simulink model "Hopper_3DOF"  (R2025a)
settings: Solver=FixedStepAuto  StartTime=0.0  StopTime=10  FixedStep=0.05  RelTol=1e-3
model workspace (MAT data in the model file):
  Inertia = 5000
  Prop_Mass = 50
libraries: aerolibanim x1
settings Model: Creator=asing  LastModifiedBy=asing

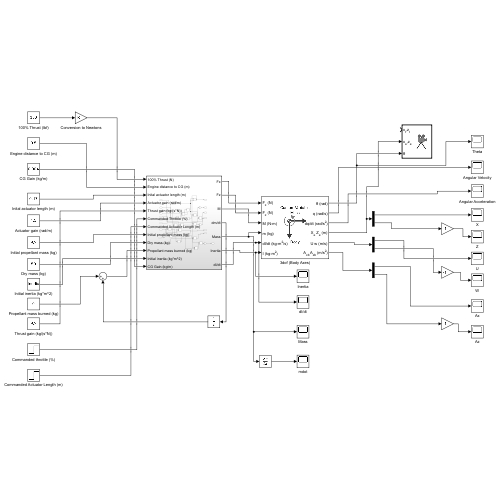
[thumbnail: Simulink's stored preview of the top-level diagram]
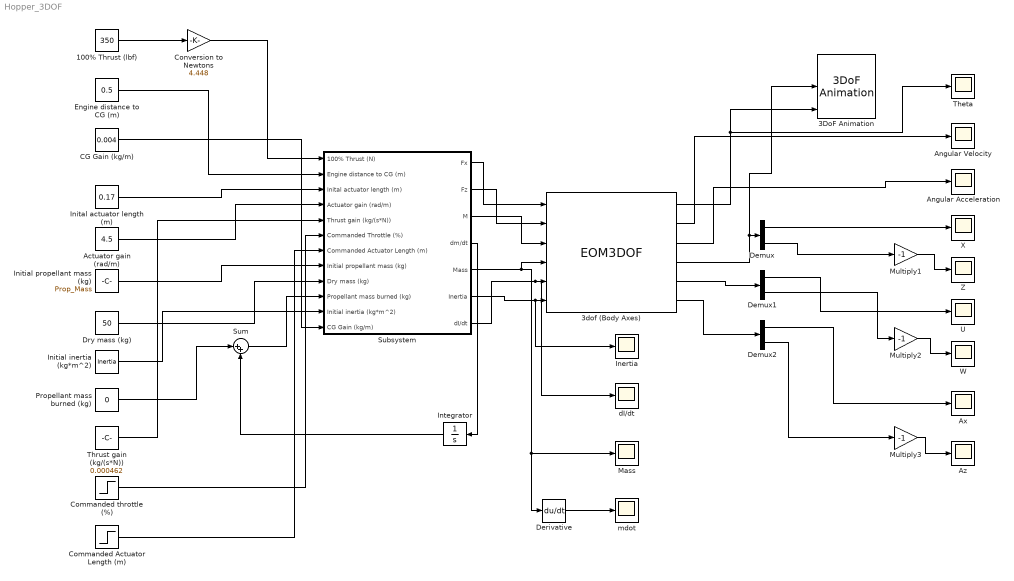
== system Hopper_3DOF ==
  100% Thrust (lbf) : Constant  Value=350
  3DoF Animation : aerolibanim/3DoF Animation  u1=[0 5000 -2000 2000 -5050 -3050]  u2=0.05  u3=1.0  u5=Fly alongside  u6=[2000 500 -3150]  u7=10  u8=on
  3dof (Body Axes) : EOM3DOF  mtype=Custom Variable  v_ini=0  mass=Mass  mass_e=50  mass_f=100  Iyy=Inertia  Iyy_e=1000  Iyy_f=5000
  Actuator gain (rad/m) : Constant  Value=4.5
  Angular Acceleration : Scope
      settings: ActiveDisplayYMinimum=0.0050078581809152025  ActiveDisplayYMaximum=0.00588060097021886  DataLoggingVariableName=ScopeData8
  Angular Velocity : Scope
      settings: ActiveDisplayYMinimum=-0.0020700029264905822  ActiveDisplayYMaximum=0.018630026338415245  DataLoggingVariableName=ScopeData3
  Ax : Scope
      settings: ActiveDisplayYMinimum=-236.39264963405441  ActiveDisplayYMaximum=707.50769830860759  DataLoggingVariableName=ScopeData6
  Az : Scope
      settings: ActiveDisplayYMinimum=1.5527082203950426  ActiveDisplayYMaximum=3.2690896985722757  DataLoggingVariableName=ScopeData7
  CG Gain (kg/m) : Constant  Value=0.004
  Commanded Actuator Length (m) : Step  Before=0.2  After=.2  SampleTime=0
  Commanded throttle (%) : Step  Before=1  SampleTime=0
  Conversion to Newtons : Gain  Gain=4.448
  Demux : Demux  Outputs=2
  Demux1 : Demux  Outputs=2
  Demux2 : Demux  Outputs=2
  Derivative : Derivative
  Dry mass (kg) : Constant  Value=50
  Engine distance to CG (m) : Constant  Value=0.5
  Inertia : Scope
      settings: ActiveDisplayYMinimum=4535.2486810070413  ActiveDisplayYMaximum=5055.6312167570431  DataLoggingVariableName=ScopeData11
  Inital actuator length (m) : Constant  Value=0.17
  Initial inertia (kg*m^2) : Constant  Value=Inertia
  Initial propellant mass (kg) : Constant  Value=Prop_Mass
  Integrator : Integrator
  Mass : Scope
      settings: ActiveDisplayYMinimum=97.942983726316214  ActiveDisplayYMaximum=101.33141615987562  DataLoggingVariableName=ScopeData9
  Multiply1 : Gain  Gain=-1
  Multiply2 : Gain  Gain=-1
  Multiply3 : Gain  Gain=-1
  Propellant mass burned (kg) : Constant  Value=0
  Subsystem : Subsystem
  Sum : Sum  Inputs=|++
  Theta : Scope
      settings: ActiveDisplayYMinimum=-0.0741149748185771  ActiveDisplayYMaximum=1.4135943241841924  DataLoggingVariableName=ScopeData2
  Thrust gain (kg/(s*N)) : Constant  Value=0.000462
  U : Scope
      settings: ActiveDisplayYMinimum=-119.22167954269128  ActiveDisplayYMaximum=620.34894160906708  DataLoggingVariableName=ScopeData4
  W : Scope
      settings: ActiveDisplayYMinimum=-7.1975000000000255  ActiveDisplayYMaximum=64.777500000000245  DataLoggingVariableName=ScopeData5
  X : Scope
      settings: ActiveDisplayYMinimum=-30.09481005960259  ActiveDisplayYMaximum=270.8532905364234
  Z : Scope
      settings: ActiveDisplayYMinimum=-80.66158563219318  ActiveDisplayYMaximum=340.25793977590678
  dI/dt : Scope
      settings: ActiveDisplayYMinimum=-45.962080000000007  ActiveDisplayYMaximum=-25.962080000000007  DataLoggingVariableName=ScopeData12
  mdot : Scope
      settings: ActiveDisplayYMinimum=-0.84942705484417036  ActiveDisplayYMaximum=-0.37264058390355936  DataLoggingVariableName=ScopeData10
  wires:
  100% Thrust (lbf)/1 -> Conversion to Newtons/1
  Conversion to Newtons/1 -> Subsystem/1(100% Thrust (N))
  Engine distance to CG (m)/1 -> Subsystem/2(Engine distance to CG (m))
  Inital actuator length (m)/1 -> Subsystem/3(Inital actuator length (m))
  Actuator gain (rad/m)/1 -> Subsystem/4(Actuator gain (rad/m))
  Commanded throttle (%)/1 -> Subsystem/6(Commanded Throttle (%))
  Commanded Actuator Length (m)/1 -> Subsystem/7(Commanded Actuator Length (m))
  3dof (Body Axes)/4 -> 3DoF Animation/2, Demux/1
  Demux/1 -> X/1
  Demux/2 -> Multiply1/1
  3dof (Body Axes)/1 -> 3DoF Animation/3, Theta/1
  3dof (Body Axes)/2 -> Angular Velocity/1
  Demux1/1 -> U/1
  Demux1/2 -> Multiply2/1
  Demux2/1 -> Ax/1
  Demux2/2 -> Multiply3/1
  Multiply1/1 -> Z/1
  Multiply2/1 -> W/1
  Multiply3/1 -> Az/1
  3dof (Body Axes)/3 -> Angular Acceleration/1
  Subsystem/1(Fx) -> 3dof (Body Axes)/1
  Subsystem/2(Fz) -> 3dof (Body Axes)/2
  Subsystem/3(M) -> 3dof (Body Axes)/3
  3dof (Body Axes)/5 -> Demux1/1
  3dof (Body Axes)/6 -> Demux2/1
  Thrust gain (kg/(s*N))/1 -> Subsystem/5(Thrust gain (kg/(s*N)))
  Subsystem/5(Mass) -> Derivative/1, Mass/1, 3dof (Body Axes)/4
  Initial propellant mass (kg)/1 -> Subsystem/8(Initial propellant mass (kg))
  Initial inertia (kg*m^2)/1 -> Subsystem/11(Initial inertia (kg*m^2))
  Dry mass (kg)/1 -> Subsystem/9(Dry mass (kg))
  Integrator/1 -> Sum/2
  Propellant mass burned (kg)/1 -> Sum/1
  Sum/1 -> Subsystem/10(Propellant mass burned (kg))
  Subsystem/4(dm/dt) -> Integrator/1
  Derivative/1 -> mdot/1
  CG Gain (kg/m)/1 -> Subsystem/12(CG Gain (kg/m))
  Subsystem/6(Inertia) -> Inertia/1, 3dof (Body Axes)/6
  Subsystem/7(dI/dt) -> dI/dt/1, 3dof (Body Axes)/5

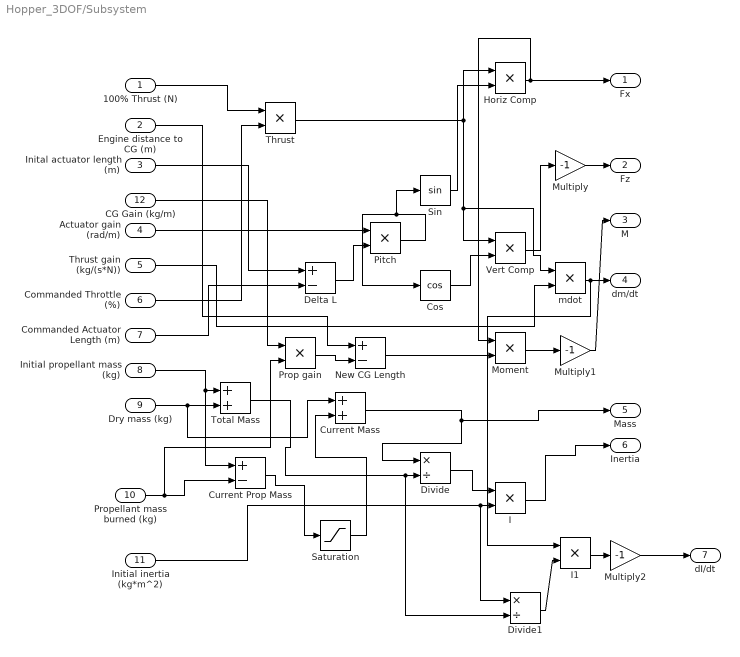
== system Hopper_3DOF/Subsystem ==
  100% Thrust (N) : Inport
  Engine distance to CG (m) : Inport  Port=2
  Inital actuator length (m) : Inport  Port=3
  Actuator gain (rad/m) : Inport  Port=4
  Thrust gain (kg/(s*N)) : Inport  Port=5
  Commanded Throttle (%) : Inport  Port=6
  Commanded Actuator Length (m) : Inport  Port=7
  Initial propellant mass (kg) : Inport  Port=8
  Dry mass (kg) : Inport  Port=9
  Propellant mass burned (kg) : Inport  Port=10
  Initial inertia (kg*m^2) : Inport  Port=11
  CG Gain (kg/m) : Inport  Port=12
  Cos : Trigonometry  Operator=cos
  Current Mass : Sum
  Current Prop Mass : Sum  Inputs=+-
  Delta L : Sum  Inputs=+-
  Divide : Product  Inputs=*/
  Divide1 : Product  Inputs=*/
  Horiz Comp : Product
  I : Product
  I1 : Product
  Moment : Product
  Multiply : Gain  Gain=-1
  Multiply1 : Gain  Gain=-1
  Multiply2 : Gain  Gain=-1
  New CG Length : Sum  Inputs=+-
  Pitch : Product
  Prop gain : Product
  Saturation : Saturate  UpperLimit=Prop_Mass  LowerLimit=0
  Sin : Trigonometry
  Thrust : Product
  Total Mass : Sum
  Vert Comp : Product
  mdot : Product
  Fx : Outport
  Fz : Outport  Port=2
  M : Outport  Port=3
  dm/dt : Outport  Port=4
  Mass : Outport  Port=5
  Inertia : Outport  Port=6
  dI/dt : Outport  Port=7
  wires:
  Inital actuator length (m)/1 -> Delta L/1
  Commanded Actuator Length (m)/1 -> Delta L/2
  Delta L/1 -> Pitch/2
  Actuator gain (rad/m)/1 -> Pitch/1
  Commanded Throttle (%)/1 -> Thrust/2
  100% Thrust (N)/1 -> Thrust/1
  Pitch/1 -> Cos/1, Sin/1
  Sin/1 -> Horiz Comp/2
  Thrust/1 -> Vert Comp/1, mdot/1, Horiz Comp/1
  Horiz Comp/1 -> Moment/1, Fx/1
  Cos/1 -> Vert Comp/2
  Moment/1 -> Multiply1/1
  Multiply/1 -> Fz/1
  Multiply1/1 -> M/1
  Vert Comp/1 -> Multiply/1
  Thrust gain (kg/(s*N))/1 -> mdot/2
  Propellant mass burned (kg)/1 -> Prop gain/2, Current Prop Mass/2
  Divide/1 -> I/1
  Initial inertia (kg*m^2)/1 -> Divide1/1, I/2
  I/1 -> Inertia/1
  Current Mass/1 -> Divide/1, Mass/1
  Initial propellant mass (kg)/1 -> Current Prop Mass/1, Total Mass/1
  Dry mass (kg)/1 -> Current Mass/1, Total Mass/2
  Total Mass/1 -> Divide1/2, Divide/2
  Current Prop Mass/1 -> Saturation/1
  Saturation/1 -> Current Mass/2
  mdot/1 -> I1/1, dm/dt/1
  Multiply2/1 -> dI/dt/1
  CG Gain (kg/m)/1 -> Prop gain/1
  Engine distance to CG (m)/1 -> New CG Length/1
  Prop gain/1 -> New CG Length/2
  New CG Length/1 -> Moment/2
  Divide1/1 -> I1/2
  I1/1 -> Multiply2/1
